simulink model "Computed_Torque"  (R2021a)
settings: Solver=VariableStepAuto  StartTime=0.0  StopTime=10  RelTol=1e-3
values from neighbouring files (symbols this model uses):
  Exp1 = K_P*K_V*K_A*T_A+K_V*k_TP*K_A/k_TP    [param_Computed_Torque.m]
  Exp2 = K_P*K_V*K_A    [param_Computed_Torque.m]
  Exp3 = (K_V*k_TV*K_A*T_A+K_A*k_TA)/k_TP    [param_Computed_Torque.m]
  Exp4 = K_A*T_A*k_TA/k_TP    [param_Computed_Torque.m]
  F_v = zeros(6,6)    [param_Computed_Torque.m]
  k_m = 1/k_v    (= 2)    [param_Computed_Torque.m]
  K_R = diag(k_r)    [param_Computed_Torque.m]
  K_T = 15*eye(6,6)    [param_Computed_Torque.m]
  k_TP = eye(6,6)    [param_Computed_Torque.m]
  q_i = zeros(6,1)    [param_Computed_Torque.m]
  R_a = 2*eye(6,6)    [param_Computed_Torque.m]
  T_m = Im    [param_Computed_Torque.m]
settings Model: OrderedModelArguments=off  Creator=ASUS  LastModifiedBy=Nikunj Sanghai
settings SolverCC: AlgebraicLoopSolver=TrustRegion

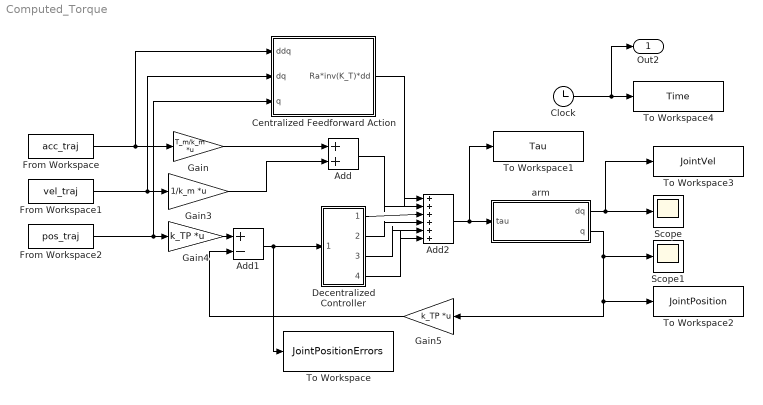
== system Computed_Torque ==
  "\tCentralized Feedforward Action" : Subsystem
  Add : Sum
  Add1 : Sum  Inputs=+-
  Add2 : Sum  Inputs=++++++
  Clock : Clock
  Decentralized Controller : Subsystem
  From Workspace : FromWorkspace  VariableName=acc_traj  OutputAfterFinalValue=Holding final value
  From Workspace1 : FromWorkspace  VariableName=vel_traj  OutputAfterFinalValue=Holding final value
  From Workspace2 : FromWorkspace  VariableName=pos_traj  OutputAfterFinalValue=Holding final value
  Gain : Gain  Gain=T_m/k_m  Multiplication=Matrix(K*u)
  Gain3 : Gain  Gain=1/k_m  Multiplication=Matrix(K*u)
  Gain4 : Gain  Gain=k_TP  Multiplication=Matrix(K*u)
  Gain5 : Gain  Gain=k_TP  Multiplication=Matrix(K*u)
  Scope : Scope
  Scope1 : Scope
  To Workspace : ToWorkspace  VariableName=JointPositionErrors  SaveFormat=Timeseries  SampleTime=-1
  To Workspace1 : ToWorkspace  VariableName=Tau  SaveFormat=Timeseries  SampleTime=-1
  To Workspace2 : ToWorkspace  VariableName=JointPosition  SaveFormat=Timeseries  SampleTime=-1
  To Workspace3 : ToWorkspace  VariableName=JointVel  SaveFormat=Timeseries  SampleTime=-1
  To Workspace4 : ToWorkspace  VariableName=Time  SaveFormat=Timeseries  SampleTime=-1
  arm : Subsystem
      mask Display: disp('inv(B(q))(tau-tau'')')
  Out2 : Outport
  wires:
  From Workspace/1 -> "\tCentralized Feedforward Action"/1(ddq), Gain/1
  From Workspace1/1 -> Gain3/1, "\tCentralized Feedforward Action"/2(dq)
  Gain/1 -> Add/1
  Gain3/1 -> Add/2
  From Workspace2/1 -> "\tCentralized Feedforward Action"/3(q), Gain4/1
  Gain4/1 -> Add1/1
  Gain5/1 -> Add1/2
  Add1/1 -> To Workspace/1, Decentralized Controller/1(In1)
  arm/2("q ") -> Scope1/1, To Workspace2/1, Gain5/1
  arm/1(dq) -> Scope/1, To Workspace3/1
  Add2/1 -> arm/1(tau), To Workspace1/1
  Clock/1 -> Out2/1, To Workspace4/1
  Add/1 -> Add2/2
  "\tCentralized Feedforward Action"/1(Ra*inv(K_T)*dd) -> Add2/1
  Decentralized Controller/1(Out1) -> Add2/3
  Decentralized Controller/2(Out2) -> Add2/4
  Decentralized Controller/3(Out3) -> Add2/5
  Decentralized Controller/4(Out4) -> Add2/6

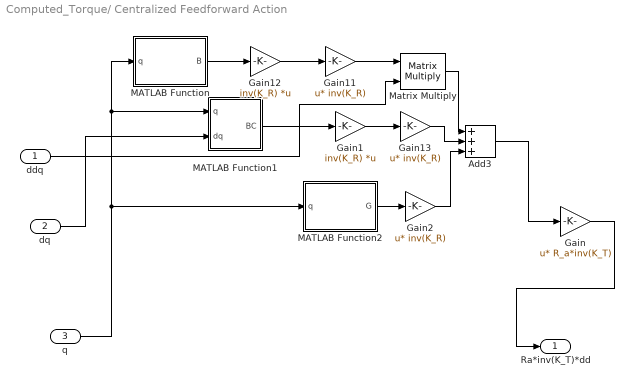
== system Computed_Torque/	Centralized Feedforward Action ==
  ddq : Inport
  dq : Inport  Port=2
  q : Inport  Port=3
  Add3 : Sum  Inputs=+++
  Gain : Gain  Gain=R_a*inv(K_T)  Multiplication=Matrix(u*K)
  Gain1 : Gain  Gain=inv(K_R)  Multiplication=Matrix(K*u)
  Gain11 : Gain  Gain=inv(K_R)  Multiplication=Matrix(u*K)
  Gain12 : Gain  Gain=inv(K_R)  Multiplication=Matrix(K*u)
  Gain13 : Gain  Gain=inv(K_R)  Multiplication=Matrix(u*K)
  Gain2 : Gain  Gain=inv(K_R)  Multiplication=Matrix(u*K)
  MATLAB Function : MATLAB Function  TreatAsAtomicUnit=on
  MATLAB Function1 : MATLAB Function  TreatAsAtomicUnit=on
  MATLAB Function2 : MATLAB Function  TreatAsAtomicUnit=on
  Matrix Multiply : Product  Multiplication=Matrix(*)
  Ra*inv(K_T)*dd : Outport
  wires:
  Gain12/1 -> Gain11/1
  Gain13/1 -> Add3/2
  Gain11/1 -> Matrix Multiply/1
  MATLAB Function1/1(BC) -> Gain1/1
  Gain1/1 -> Gain13/1
  Matrix Multiply/1 -> Add3/1
  MATLAB Function/1(B) -> Gain12/1
  q/1 -> MATLAB Function1/1(q), MATLAB Function/1(q), MATLAB Function2/1(q)
  dq/1 -> MATLAB Function1/2(dq)
  ddq/1 -> Matrix Multiply/2
  MATLAB Function2/1(G) -> Gain2/1
  Gain2/1 -> Add3/3
  Add3/1 -> Gain/1
  Gain/1 -> Ra*inv(K_T)*dd/1

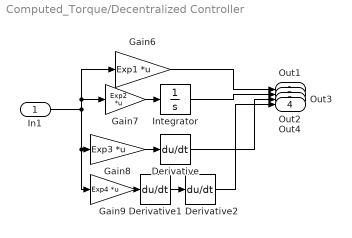
== system Computed_Torque/Decentralized Controller ==
  In1 : Inport
  Derivative : Derivative  CoefficientInTFapproximation=0
  Derivative1 : Derivative  CoefficientInTFapproximation=0
  Derivative2 : Derivative  CoefficientInTFapproximation=0
  Gain6 : Gain  Gain=Exp1  Multiplication=Matrix(K*u)
  Gain7 : Gain  Gain=Exp2  Multiplication=Matrix(K*u)
  Gain8 : Gain  Gain=Exp3  Multiplication=Matrix(K*u)
  Gain9 : Gain  Gain=Exp4  Multiplication=Matrix(K*u)
  Integrator : Integrator  InitialCondition=[0 0 0 0 0 0]'
  Out1 : Outport
  Out2 : Outport  Port=2
  Out3 : Outport  Port=3
  Out4 : Outport  Port=4
  wires:
  Gain8/1 -> Derivative/1
  Gain6/1 -> Out1/1
  Gain9/1 -> Derivative1/1
  Gain7/1 -> Integrator/1
  In1/1 -> Gain6/1, Gain7/1, Gain9/1, Gain8/1
  Derivative1/1 -> Derivative2/1
  Integrator/1 -> Out2/1
  Derivative2/1 -> Out4/1
  Derivative/1 -> Out3/1

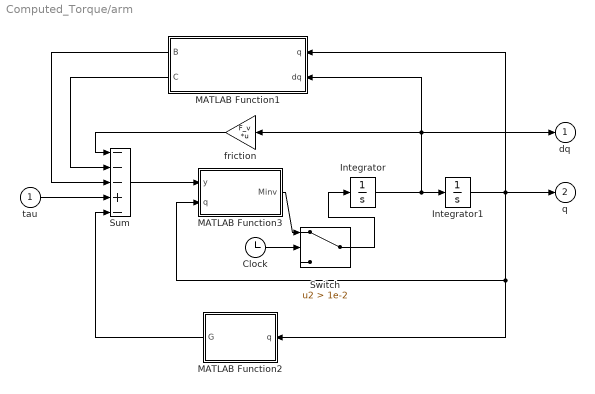
== system Computed_Torque/arm ==
  tau : Inport
  Clock : Clock
  Integrator : Integrator  InitialCondition=[0 0 0 0 0 0]'  ZeroCross=off
  Integrator1 : Integrator  InitialCondition=q_i  ZeroCross=off
  MATLAB Function1 : MATLAB Function  TreatAsAtomicUnit=on
  MATLAB Function2 : MATLAB Function  TreatAsAtomicUnit=on
  MATLAB Function3 : MATLAB Function  TreatAsAtomicUnit=on
  Sum : Sum  Inputs=---+-  InputSameDT=on  SaturateOnIntegerOverflow=on  OutDataTypeStr=Inherit: Same as first input
  Switch : Switch  Criteria=u2 > Threshold  Threshold=1e-2
  friction : Gain  Gain=F_v  Multiplication=Matrix(K*u)  SaturateOnIntegerOverflow=on  OutDataTypeStr=Inherit: Same as input  ParamDataTypeStr=Inherit: Same as input
      mask Display: disp('F_v')
  dq : Outport  InitialOutput=0
  "q " : Outport  Port=2  InitialOutput=0
  wires:
  Integrator1/1 -> MATLAB Function3/2(q), MATLAB Function2/1(q), MATLAB Function1/1(q), "q "/1
  Integrator/1 -> Integrator1/1, friction/1, MATLAB Function1/2(dq), dq/1
  Sum/1 -> MATLAB Function3/1(y)
  friction/1 -> Sum/1
  MATLAB Function2/1(G) -> Sum/5
  tau/1 -> Sum/4
  MATLAB Function1/1(B) -> Sum/3
  MATLAB Function1/2(C) -> Sum/2
  Clock/1 -> Switch/2
  Switch/1 -> Integrator/1
  MATLAB Function3/1(Minv) -> Switch/1

== matlab function Computed_Torque/	Centralized Feedforward Action/MATLAB Function ==
  data: q input; B output
function B = inertia(q)
B=inertia(q);
end

== matlab function Computed_Torque/arm/MATLAB Function1 ==
  data: q input; B output; dq input; C output
function [B,C] = corioliscentrifugalsim(q, dq)
[B,C] = corioliscentrifugal(q, dq);
end

== matlab function Computed_Torque/arm/MATLAB Function2 ==
  data: q input; G output
function G = gravitysim(q)
G = gravity(q);
end

== matlab function Computed_Torque/arm/MATLAB Function3 ==
  data: y input; q input; Minv output
function Minv = inertiainvsim(y, q)
M = inertia(q);
% M=M(1:3,1:3);
Minv = inv(M)*y;

end

== matlab function Computed_Torque/	Centralized Feedforward Action/MATLAB Function2 ==
  data: q input; G output
function G = gravity(q)
G=gravity(q);
end

== matlab function Computed_Torque/	Centralized Feedforward Action/MATLAB Function1 ==
  data: q input; BC output; dq input
function BC  = corioliscentrifugal(q,dq)
[B,C]=corioliscentrifugal(q,dq);
BC=B+C;
end
